simulink model "Auxiliaries_Torque_Sum"  (R2016b)
settings: Solver=FixedStepDiscrete  StartTime=0.0  StopTime=inf  FixedStep=AuxTqSum.tiSimnTiStep_C.Value  RelTol=1e-3  EnableMultiTasking=on
settings Model: Creator=djuenema  LastModifiedBy=djuenema
settings DataIOCC: SaveFormat=StructureWithTime  SaveOutput=off  DSMLogging=off  VisualizeSimOutput=off  SaveTime=off  SignalLoggingName=Results
settings OptimizationCC: BlockReduction=off  ConditionallyExecuteInputs=off  LifeSpan=inf
settings DebuggingCC: AllowSymbolicDim=off  SFUnexpectedBacktrackingDiag=warning  SFNoUnconditionalDefaultTransitionDiag=warning  SFExecutionAtInitializationDiag=none
settings ModelReferenceCC: ModelReferenceNumInstancesAllowed=Single  PropagateSignalLabelsOutOfModel=off
settings GRTTargetCC: TargetLangStandard=C89/C90 (ANSI)
settings ConfigComp: CovMetricSettings=dw  CovHtmlReporting=on  CovSaveCumulativeToWorkspaceVar=on  CovSaveSingleToWorkspaceVar=on  CovExternalEMLEnable=off

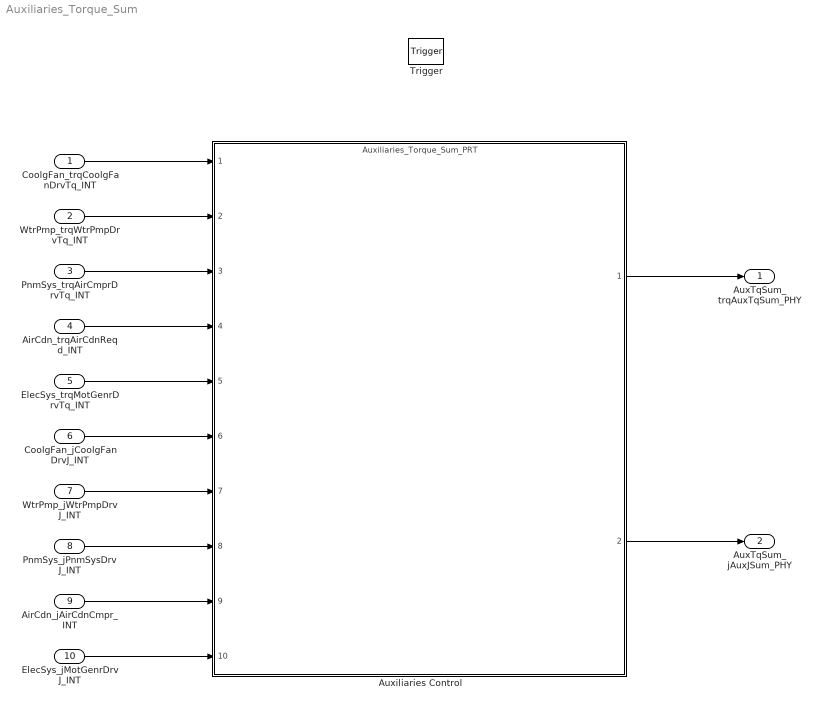
== system Auxiliaries_Torque_Sum ==
  CoolgFan_trqCoolgFanDrvTq_INT : Inport
  WtrPmp_trqWtrPmpDrvTq_INT : Inport  Port=2
  PnmSys_trqAirCmprDrvTq_INT : Inport  Port=3
  AirCdn_trqAirCdnReqd_INT : Inport  Port=4
  ElecSys_trqMotGenrDrvTq_INT : Inport  Port=5
  CoolgFan_jCoolgFanDrvJ_INT : Inport  Port=6
  WtrPmp_jWtrPmpDrvJ_INT : Inport  Port=7
  PnmSys_jPnmSysDrvJ_INT : Inport  Port=8
  AirCdn_jAirCdnCmpr_INT : Inport  Port=9
  ElecSys_jMotGenrDrvJ_INT : Inport  Port=10
  Trigger : TriggerPort  TriggerType=function-call  VariantControl=Variant  PortDimensions=1
  Auxiliaries Control : ModelReference  ModelNameDialog=Auxiliaries_Torque_Sum_PRT.slxp  ModelReferenceVersion=1.3  CopyOfModelProtected=on
  AuxTqSum_trqAuxTqSum_PHY : Outport
  AuxTqSum_jAuxJSum_PHY : Outport  Port=2
  wires:
  Auxiliaries Control/2 -> AuxTqSum_jAuxJSum_PHY/1
  Auxiliaries Control/1 -> AuxTqSum_trqAuxTqSum_PHY/1
  WtrPmp_trqWtrPmpDrvTq_INT/1 -> Auxiliaries Control/2
  PnmSys_trqAirCmprDrvTq_INT/1 -> Auxiliaries Control/3
  CoolgFan_trqCoolgFanDrvTq_INT/1 -> Auxiliaries Control/1
  AirCdn_trqAirCdnReqd_INT/1 -> Auxiliaries Control/4
  ElecSys_trqMotGenrDrvTq_INT/1 -> Auxiliaries Control/5
  CoolgFan_jCoolgFanDrvJ_INT/1 -> Auxiliaries Control/6
  WtrPmp_jWtrPmpDrvJ_INT/1 -> Auxiliaries Control/7
  PnmSys_jPnmSysDrvJ_INT/1 -> Auxiliaries Control/8
  AirCdn_jAirCdnCmpr_INT/1 -> Auxiliaries Control/9
  ElecSys_jMotGenrDrvJ_INT/1 -> Auxiliaries Control/10
